simulink model "HelicopterProject"  (R2023b)
settings: Solver=ode4  StartTime=0.0  StopTime=20  FixedStep=0.002  RelTol=1e-3  EnableMultiTasking=on
InitFcn:
  | % NOTE: If using VoltPAQ-X1, make sure both Gain switches are set to 3.
  | K_AMP = 3;
  | 
  | % Maximum Output Voltage (V): YAW limited to 15 V. PITCH limited to 24 V.
  | VMAX_AMP_P = 24;
  | VMAX_AMP_Y = 15;
  | 
  | % Initial Angle of Pitch (rad)
  | theta_0 = 10*pi/180;
  | phsy_0 = -10*pi/180;
  | 
  | % Performance specifications
  | settle_range_p = 0.003;
  | rise_range_theta_low = 0.1 * theta_0;
  | rise_range_theta_up = 0.9 * theta_0;
  | 
  | rise_range_phsy_low = 0.1 * phsy_0;
  | rise_range_phsy_up = 0.9 * phsy_0;
  | 
  | 
  | g = 9.81;
  | 
  | % Pitch and Yaw Motor Voltage-Torque Constant (N.m/V)
  | % The amount of torque the motor generates per unit of input V   !!
  | K_yp = 0.0219;
  | K_py = 0.0068;
  | 
  | % Pitch and Yaw Viscous Damping Constant (N.m.s/rad)
  | B_p = 0.8;
  | B_y = 0.318;
  | 
  | % Mass of the Helicopter (kg)
  | m = 1.3872;
  | 
  | % Pitch and Yaw Propeller Torque-Thrust Constant found Experimentally (N.m/V)
  | % how much rotational torque is generated by the trust applied on each
  | % motor. Depends on the distance of the point where the trust is applied.
  | % !!
  | K_pp = 0.204;
  | K_yy = 0.072;
  | 
  | % Helicopter Center of Mass from Pivot along Pitch Axis (m)
  | l = 0.186;
  | 
  | J_eq_p = 0.0384;
  | J_eq_y = 0.0432;
  | 
  | A=[      0         0      1.0000                  0
  |          0         0         0                 1.0000
  |          0         0   -B_p/(J_eq_p+m*l^2)        0
  |          0         0         0             -B_y/(J_eq_y+m*l^2)];
  | 
  | B=[      0                     0
  |          0                     0
  |     K_pp/(J_eq_p+m*l^2)   K_py/(J_eq_p+m*l^2)
  |     K_yp/(J_eq_y+m*l^2)   K_yy/(J_eq_y+m*l^2)];
  | 
  | 
  | Q =[35 0 0 0; 0 35 0 0; 0 0 1 0; 0 0 0 1];
  | %Q = eye(4);
  | R = [1 0; 0 1];
  | K = lqr(A,B,Q,R);
  | 
  | u2_star = m*g*l/(K_py - K_pp*K_yy/K_yp);
  | u1_star = -(K_yy * u2_star)/K_yp ;
  | 
  | 
  | % Bessel gains
  | Kbes=[     68.5119  -25.1203    5.3421   -3.6881
  |    63.1652  188.4894    0.7783   19.4789];
settings Model: ExtModeTrigDuration=10000  Creator=Sona  LastModifiedBy=Sona
settings SolverCC: AlgebraicLoopSolver=TrustRegion  PositivePriorityOrder=on
settings DataIOCC: ReturnWorkspaceOutputs=off
settings DebuggingCC: UnconnectedInputMsg=warning  UnconnectedOutputMsg=warning  UnconnectedLineMsg=warning  ArithmeticOperatorsInVariantConditions=warning
settings ModelReferenceCC: EnableRefExpFcnMdlSchedulingChecks=on
settings SFSimCC: SimUseLocalCustomCode=off  CustomCodeUndefinedFunction=UseInterfaceOnly
settings RTWCC: Description=QUARC Win64 Target Using Toolchain  SystemTargetFile=quarc_win64.tlc  TemplateMakefile=quarc_default_tmf  RTWUseLocalCustomCode=off  Toolchain=QUARC win64 | nmake (64-bit Windows)  BuildConfiguration=Faster Runs
settings CodeAppCC: StateflowObjectComments=on
settings STFCustomTargetCC: ConcurrentExecutionCompliant=on  GRTInterface=on  UseToolchainInfoCompliant=on  SystemTargetFile=quarc_win64.tlc
settings GRTTargetCC: ParMdlRefBuildCompliant=off  CompOptLevelCompliant=off  CombineOutputUpdateFcns=off  MatFileLogging=off  CPPClassGenCompliant=off  GRTInterface=on  ExtMode=on  ExtModeMexFile=quarc_comm
settings ConfigComp: CovMetricSettings=dswe

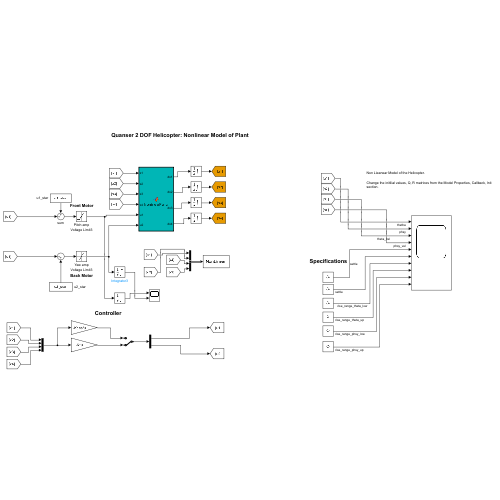
[thumbnail: Simulink's stored preview of the top-level diagram]
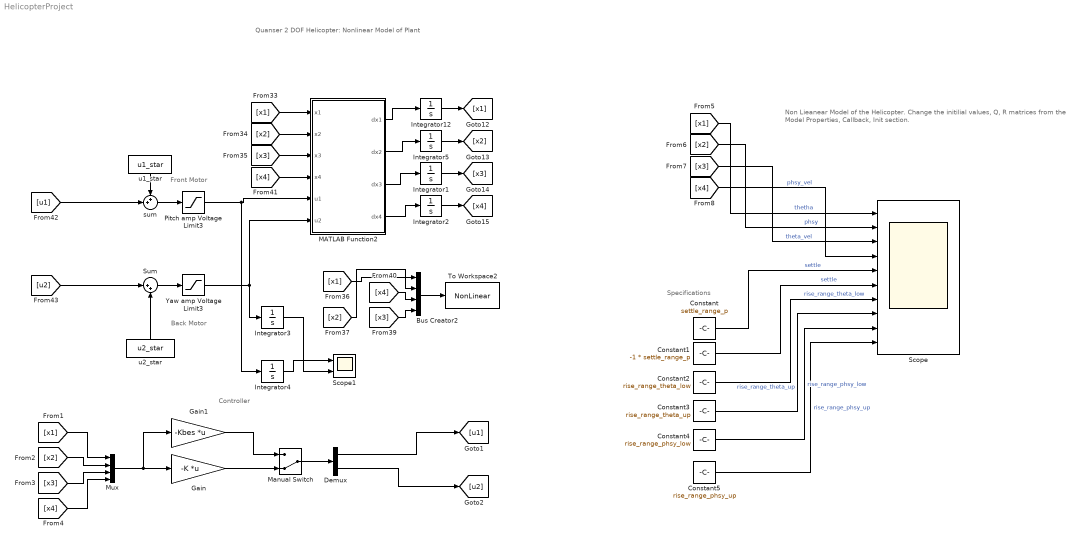
== system HelicopterProject ==
  note: Non Lieanear Model of the Helicopter.
      |
      | Change the initilial values, Q, R matrices from the Model Properties, Callback, Init
      | section.
  note: Quanser 2 DOF Helicopter: Nonlinear Model of Plant
  note: Back Motor
  note: Front Motor
  note: Controller
  note: Specifications
  Bus Creator2 : BusCreator  Inputs=4
  Constant : Constant  Value=settle_range_p
  Constant1 : Constant  Value=-1 * settle_range_p
  Constant2 : Constant  Value=rise_range_theta_low
  Constant3 : Constant  Value=rise_range_theta_up
  Constant4 : Constant  Value=rise_range_phsy_low
  Constant5 : Constant  Value=rise_range_phsy_up
  Demux : Demux  Outputs=2
  Gain : Gain  Gain=-K  Multiplication=Matrix(K*u)
  Gain1 : Gain  Gain=-Kbes  Multiplication=Matrix(K*u)
  Integrator1 : Integrator  InitialCondition=0.20  LimitOutput=on  UpperSaturationLimit=0.25  LowerSaturationLimit=-0.25
  Integrator12 : Integrator  InitialCondition=theta_0  LimitOutput=on  UpperSaturationLimit=10 * pi/180  LowerSaturationLimit=-10*pi/180
  Integrator2 : Integrator  InitialCondition=-0.20  LimitOutput=on  UpperSaturationLimit=0.25  LowerSaturationLimit=-0.25
  Integrator3 : Integrator  InitialCondition=0.2  LimitOutput=on  UpperSaturationLimit=0.25  LowerSaturationLimit=-0.25
  Integrator4 : Integrator  InitialCondition=0.2  LimitOutput=on  UpperSaturationLimit=0.25  LowerSaturationLimit=-0.25
  Integrator5 : Integrator  InitialCondition=phsy_0  LimitOutput=on  UpperSaturationLimit=10*pi/180  LowerSaturationLimit=-10*pi/180
  MATLAB Function2 : MATLAB Function  TreatAsAtomicUnit=on
  Manual Switch : ManualSwitch  CurrentSetting=0
  Mux : Mux
  Pitch amp Voltage Limit3 : Saturate  UpperLimit=VMAX_AMP_P  LowerLimit=- VMAX_AMP_P
  Scope : Scope  NumInputPorts=10
  Scope1 : Scope  NumInputPorts=2
  Sum : Sum  Inputs=|++
  To Workspace2 : ToWorkspace  VariableName=NonLinear  SampleTime=-1
  Yaw amp Voltage Limit3 : Saturate  UpperLimit=VMAX_AMP_Y  LowerLimit=- VMAX_AMP_Y
  sum : Sum  Inputs=++|
  u1_star : Constant  Value=u1_star
  u2_star : Constant  Value=u2_star
  wires:
  Pitch amp Voltage Limit3/1 -> Integrator4/1, MATLAB Function2/5(u1)
  Yaw amp Voltage Limit3/1 -> Integrator3/1, MATLAB Function2/6(u2)
  [x4] -> MATLAB Function2/4(x4)
  Integrator2/1 -> [x4]
  MATLAB Function2/1(dx1) -> Integrator12/1
  [u2] -> Sum/1
  [x2] -> MATLAB Function2/2(x2)
  Integrator12/1 -> [x1]
  MATLAB Function2/3(dx3) -> Integrator1/1
  [x3] -> Bus Creator2/4
  Integrator5/1 -> [x2]
  [x2] -> Bus Creator2/2
  Integrator1/1 -> [x3]
  [x4] -> Bus Creator2/3
  Bus Creator2/1 -> To Workspace2/1
  MATLAB Function2/4(dx4) -> Integrator2/1
  [x1] -> Bus Creator2/1
  [x3] -> MATLAB Function2/3(x3)
  [x1] -> Mux/1
  [x2] -> Mux/2
  [x3] -> Mux/3
  [x4] -> Mux/4
  Mux/1 -> Gain/1, Gain1/1
  [x1] -> Scope/1  "thetha"
  [x2] -> Scope/2  "phsy"
  [x3] -> Scope/3  "theta_vel"
  [x4] -> Scope/4  "phsy_vel"
  u2_star/1 -> Sum/2
  Sum/1 -> Yaw amp Voltage Limit3/1
  sum/1 -> Pitch amp Voltage Limit3/1
  [u1] -> sum/2
  u1_star/1 -> sum/1
  Demux/1 -> [u1]
  Gain1/1 -> Manual Switch/1
  Gain/1 -> Manual Switch/2
  Manual Switch/1 -> Demux/1
  Constant/1 -> Scope/5  "settle"
  Constant1/1 -> Scope/6  "settle"
  Constant2/1 -> Scope/7  "rise_range_theta_low"
  Constant3/1 -> Scope/8  "rise_range_theta_up"
  Constant4/1 -> Scope/9  "rise_range_phsy_low"
  Constant5/1 -> Scope/10  "rise_range_phsy_up"
  [x1] -> MATLAB Function2/1(x1)
  MATLAB Function2/2(dx2) -> Integrator5/1
  Demux/2 -> [u2]
  Integrator3/1 -> Scope1/2
  Integrator4/1 -> Scope1/1

== matlab function HelicopterProject/MATLAB Function2 ==
  data: x1 input; x2 input; x3 input; x4 input; u1 input; dx1 output; u2 input; dx2 output; dx3 output; dx4 output
function [dx1,dx2,dx3,dx4]= NonlinearFunc(x1,x2,x3,x4,u1,u2)
%% Initial Conditions
% Gravitational Constant (m/s^2)
g = 9.81;

% Pitch and Yaw Motor Voltage-Torque Constant (N.m/V)
% The amount of torque the motor generates per unit of input V   !!
K_yp = 0.0219;
K_py = 0.0068;

% Pitch and Yaw Viscous Damping Constant (N.m.s/rad)
B_p = 0.8; 
B_y = 0.318; 

% Mass of the Helicopter (kg)
m = 1.3872;

% Pitch and Yaw Propeller Torque-Thrust Constant found Experimentally (N.m/V)
% how much rotational torque is generated by the trust applied on each
% motor. Depends on the distance of the point where the trust is applied.
% !!
K_pp = 0.204;
K_yy = 0.072;

% Helicopter Center of Mass from Pivot along Pitch Axis (m)
l = 0.186;

J_eq_p = 0.0384;
J_eq_y = 0.0432;
%%
%%

dx1=x3;
dx2=x4;
dx3=(1/(J_eq_p +m*l^2))*((K_pp*u1+K_py*u2)-(B_p*x3+m*l^2*x4^2*sin(x1)*cos(x1)+m*g*l*cos(x1)));
dx4=1/(J_eq_y + m*l^2* (cos(x1))^2 ) * (((K_yp*u1 )+(K_yy*u2 ))-B_y*x4+2*m*l^2*x4*x3*sin(x1)*cos(x1));
